simulink model "Example"  (R2024b)
settings: Solver=VariableStepAuto  StartTime=0.0  StopTime=10.0  RelTol=1e-3
settings Model: Creator=saijaz  LastModifiedBy=saijaz

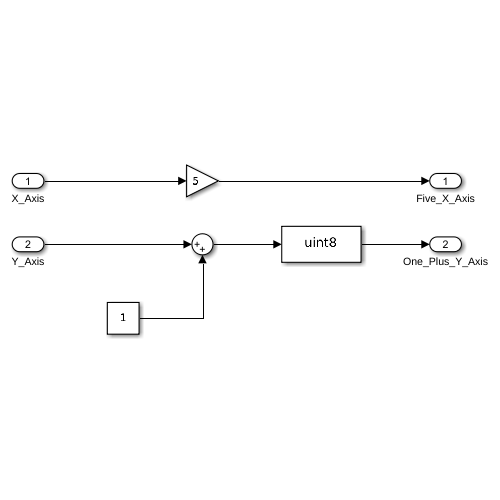
[thumbnail: Simulink's stored preview of the top-level diagram]
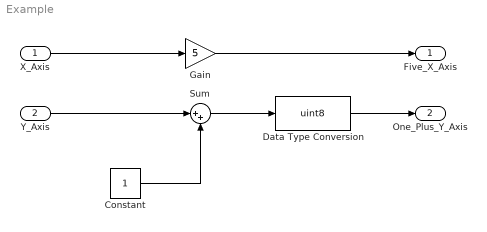
== system Example ==
  X_Axis : Inport  OutDataTypeStr=double
  Y_Axis : Inport  Port=2  OutDataTypeStr=double
  Constant : Constant  OutDataTypeStr=double
  Data Type Conversion : DataTypeConversion  OutDataTypeStr=uint8  SaturateOnIntegerOverflow=off  RndMeth=Floor
  Gain : Gain  Gain=5
  Sum : Sum  Inputs=|++
  Five_X_Axis : Outport
  One_Plus_Y_Axis : Outport  Port=2  OutDataTypeStr=uint8
  wires:
  X_Axis/1 -> Gain/1
  Gain/1 -> Five_X_Axis/1
  Constant/1 -> Sum/2
  Y_Axis/1 -> Sum/1
  Sum/1 -> Data Type Conversion/1
  Data Type Conversion/1 -> One_Plus_Y_Axis/1
